simulink model "Cuarto"  (R2017b)
settings: Solver=VariableStepAuto  StartTime=0.0  StopTime=10.0  RelTol=1e-3
settings Model: Creator=Cx001la  LastModifiedBy=Cx001la

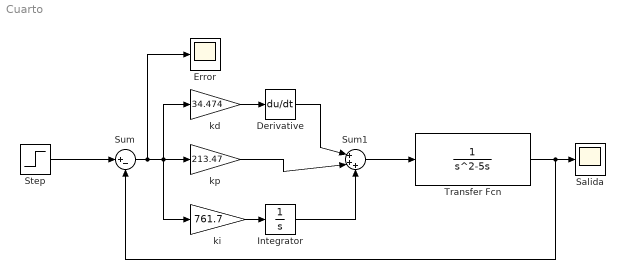
== system Cuarto ==
  Derivative : Derivative
  Error : Scope
  Integrator : Integrator
  Salida : Scope
  Step : Step  Time=0  SampleTime=0
  Sum : Sum  Inputs=|+-
  Sum1 : Sum  Inputs=|+++
  Transfer Fcn : TransferFcn  Denominator=[1 -5 0]
  kd : Gain  Gain=34.474
  ki : Gain  Gain=761.7
  kp : Gain  Gain=213.47
  wires:
  Step/1 -> Sum/1
  Sum/1 -> Error/1, ki/1, kd/1, kp/1
  kd/1 -> Derivative/1
  ki/1 -> Integrator/1
  Derivative/1 -> Sum1/1
  kp/1 -> Sum1/2
  Integrator/1 -> Sum1/3
  Sum1/1 -> Transfer Fcn/1
  Transfer Fcn/1 -> Sum/2, Salida/1
